simulink model "PeakCurrentFullBridge"  (R2021a)
settings: Solver=VariableStepAuto  StartTime=0.0  StopTime=0.02  RelTol=1e-3
libraries: spsMosfetLib x4, spsSeriesRLCBranchLib x3, spsCurrentMeasurementLib x2, spsDCVoltageSourceLib x1, simulink x1, spsSawtoothGeneratorLib x1, eeGeneralControl x1, spspowerguiLib x1
settings Model: Creator=Damian  LastModifiedBy=Damian

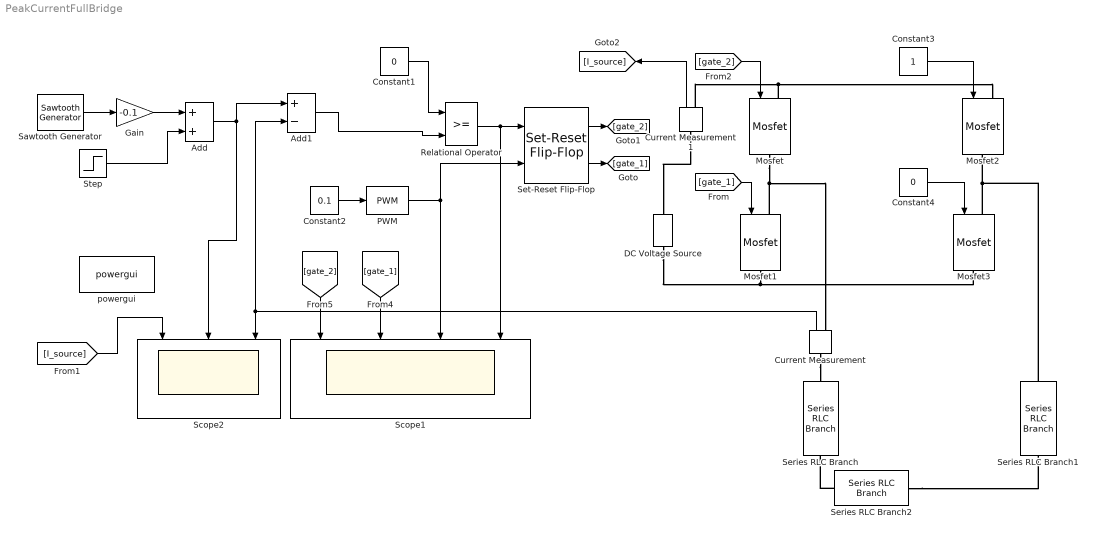
== system PeakCurrentFullBridge ==
  Add : Sum
  Add1 : Sum  Inputs=+-
  Constant1 : Constant  Value=0
  Constant2 : Constant  Value=0.1
  Constant3 : Constant
  Constant4 : Constant  Value=0
  Current Measurement : spsCurrentMeasurementLib/Current Measurement  PhasorSimulation=off  OutputType=Complex  PSBequivalent=0
  Current Measurement1 : spsCurrentMeasurementLib/Current Measurement  PhasorSimulation=off  OutputType=Complex  PSBequivalent=0
  DC Voltage Source : spsDCVoltageSourceLib/DC Voltage Source  Amplitude=100  Measurements=None
  Gain : Gain  Gain=-0.1
  Mosfet{,1..3} (4 alike) : spsMosfetLib/Mosfet  Ron=0.1  Lon=0  Rd=0.01  Vfd=0  IC=0  Rs=1e5  Cs=inf  Measurements=off
  PWM : simulink/Discontinuities/PWM  DisableCoverage=on  Period=1E-4  DisallowZeroDutyCycle=off  RunAtFixedTimeIntervals=off  SampleTime=0.1
  Relational Operator : RelationalOperator  OutDataTypeStr=boolean  RndMeth=Simplest
  Sawtooth Generator : spsSawtoothGeneratorLib/Sawtooth Generator  Freq=10e3  Phase=0  Ts=0
  Scope1 : Scope  NumInputPorts=4
  Scope2 : Scope  NumInputPorts=3
  Series RLC Branch : spsSeriesRLCBranchLib/Series RLC Branch  LConnTagsString=__new0  RConnTagsString=__new0  BranchType=L  Resistance=1  Inductance=5e-3  SetiL0=off  InitialCurrent=0  Capacitance=1e-6  Setx0=off  InitialVoltage=0  Measurements=Branch current
  Series RLC Branch1 : spsSeriesRLCBranchLib/Series RLC Branch  LConnTagsString=__new0  RConnTagsString=__new0  BranchType=L  Resistance=1  Inductance=5e-3  SetiL0=off  InitialCurrent=0  Capacitance=1e-6  Setx0=off  InitialVoltage=0  Measurements=Branch current
  Series RLC Branch2 : spsSeriesRLCBranchLib/Series RLC Branch  LConnTagsString=__new0  RConnTagsString=__new0  BranchType=R  Resistance=5  Inductance=1e-3  SetiL0=off  InitialCurrent=0  Capacitance=1e-6  Setx0=off  InitialVoltage=0  Measurements=None
  Set-Reset Flip-Flop : eeGeneralControl/Set-Reset Flip-Flop  LabelModeActiveChoice=Discrete  UndefState=Reset  Q0=0  Ts=-1
      settings: SourceProductBaseCode=PS
  Step : Step  Time=0.005  Before=9.9  After=1.9  SampleTime=0
  powergui : spspowerguiLib/powergui  Priority=1  SimulationMode=Discrete  SampleTime=1e-8  frequency=60  Iterations=50  frequencyindice=0  Pbase=100e6  ErrMax=1e-4  UnitsV=kV  UnitsW=MW  buscounter=0  FunctionMessages=off  echomessages=off  EnableUseOfTLC=off  CurrentSourceSwitches=off  DisableSnubberDevices=off  DisableRonSwitches=off  DisableVfSwitches=off  DisplayEquations=off  AutomaticDiscreteSolvers=off  SolverType=Tustin/Backward Euler (TBE)  Interpol=off  ExternalGateDelay=off  methode=off  Ts=100  x0status=blocks  SPID=on  SwTol=0  HookPort=off  NonlinearTolerance=1e-4  nMaxIteration=100  ContinueOnMaxIteration=off  RestoreLinks=warning  ResistiveCurrentMeasurement=off  Frange=[0:2:500]  Ylog=off  Xlog=on  ShowGrid=off  save=off  variable=ZData  structure=0  ZoomFFT=off  StartTime=0.0  cycles=1  DisplayStyle=1  fundamental=60  FreqAxis=off  MaxFrequency=1000  frequencyindicesteady=1  RmsSteady=1  display=off
  wires:
  Sawtooth Generator/1 -> Gain/1
  Gain/1 -> Add/1
  Step/1 -> Add/2
  Add/1 -> Scope2/2, Add1/1
  [gate_1] -> Mosfet1/1
  Constant3/1 -> Mosfet2/1
  [gate_2] -> Mosfet/1
  [gate_1] -> Scope1/2
  [gate_2] -> Scope1/1
  Current Measurement/1 -> Scope2/3, Add1/2
  Relational Operator/1 -> Set-Reset Flip-Flop/1, Scope1/4
  PWM/1 -> Set-Reset Flip-Flop/2, Scope1/3
  Constant2/1 -> PWM/1
  Constant1/1 -> Relational Operator/1
  Add1/1 -> Relational Operator/2
  Set-Reset Flip-Flop/1 -> [gate_2]
  Set-Reset Flip-Flop/2 -> [gate_1]
  Constant4/1 -> Mosfet3/1
  Current Measurement1/1 -> [I_source]
  [I_source] -> Scope2/1
  connections:
  Mosfet1/LConn1 -- Mosfet/RConn1 -- Current Measurement/RConn1
  Series RLC Branch1/LConn1 -- Mosfet3/LConn1 -- Mosfet2/RConn1
  Mosfet1/RConn1 -- DC Voltage Source/LConn1 -- Mosfet3/RConn1
  Mosfet/LConn1 -- Current Measurement1/RConn1 -- Mosfet2/LConn1
  Series RLC Branch2/LConn1 -- Series RLC Branch1/RConn1
  Series RLC Branch2/RConn1 -- Series RLC Branch/RConn1
  Current Measurement/LConn1 -- Series RLC Branch/LConn1
  Current Measurement1/LConn1 -- DC Voltage Source/RConn1
